simulink model "simuladorControlCuatrirrotor"  (Simulink 7.4)
settings: Solver=ode45  StartTime=0.0  StopTime=720  FixedStep=0.06  MaxStep=0.06  RelTol=1e-3
values from neighbouring files (symbols this model uses):
  radio = 0.1    [simulaControl.m]
  ruta = [0,0;ruta]    [pintascdata.m]    (also in pintascdata_tb2.m; simulaControl.m = [12 0;12 5;7 -5;-1 4;-6 -5;-2 0])
libraries: simulink x5
settings Model: Creator=xblasco  LastModifiedBy=xblasco

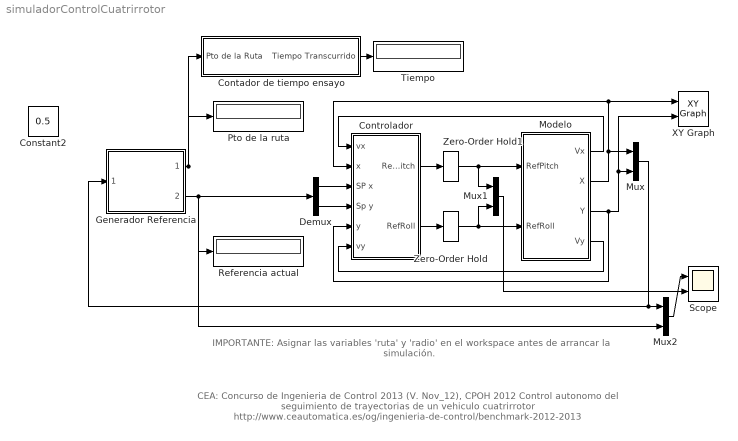
== system simuladorControlCuatrirrotor ==
  note: IMPORTANTE:
      | Asignar las variables 'ruta' y 'radio' en el workspace antes de arrancar la simulación.
  note: CEA: Concurso de Ingenieria de Control 2013 (V. Nov_12), CPOH 2012
      | Control autonomo del seguimiento de trayectorias de un vehiculo cuatrirrotor
      | http://www.ceautomatica.es/og/ingenieria-de-control/benchmark-2012-2013
  " Modelo" : Subsystem
  Contador de tiempo ensayo : Subsystem
  Controlador : Subsystem
  Demux : Demux  Outputs=2
  Generador Referencia : Subsystem
  Mux : Mux  Inputs=2
  Mux1 : Mux  Inputs=2
  Mux2 : Mux  Inputs=2
  Pto de la ruta : Display
  Referencia actual : Display
  Scope : Scope  NumInputPorts=2
      settings: YMin=-5~-1  YMax=15~1  SaveName=scdata  SampleInput=on  SampleTime=0.06
  Tiempo : Display
  XY Graph : simulink/Sinks/XY Graph  SystemSampleTime=-1  xmin=-10  xmax=15  ymin=-6  ymax=6  st=-1
  Zero-Order Hold : ZeroOrderHold  SampleTime=0.06
  Zero-Order Hold1 : ZeroOrderHold  SampleTime=0.06
  Constant2 : Constant  IOType=siggen  Value=0.5  OutDataType=sfix(16)  OutScaling=2^0
  wires:
  Generador Referencia/2(Siguiente pos) -> Referencia actual/1, Demux/1, Mux2/2
  Generador Referencia/1(Pto de la ruta) -> Pto de la ruta/1, Contador de tiempo ensayo/1(Pto de la Ruta)
  Controlador/1(RefPitch) -> Zero-Order Hold1/1
  Controlador/2(RefRoll) -> Zero-Order Hold/1
  Mux/1 -> Generador Referencia/1(Posicion  actual), Mux2/1
  Zero-Order Hold/1 -> " Modelo"/2(RefRoll), Mux1/2
  Zero-Order Hold1/1 -> " Modelo"/1(RefPitch), Mux1/1
  " Modelo"/2(X) -> Mux/1, XY Graph/1, Controlador/2(x)
  " Modelo"/3(Y) -> Controlador/5(y), XY Graph/2, Mux/2
  Mux1/1 -> Scope/2
  " Modelo"/1(Vx) -> Controlador/1(vx)
  Mux2/1 -> Scope/1
  Demux/1 -> Controlador/3(SP x)
  Demux/2 -> Controlador/4(Sp y)
  Contador de tiempo ensayo/1(Tiempo Transcurrido) -> Tiempo/1
  " Modelo"/4(Vy) -> Controlador/6(vy)

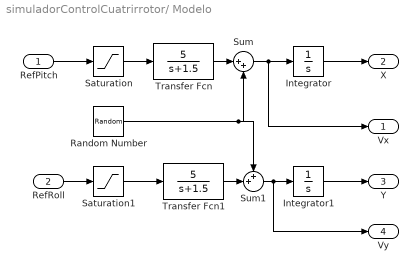
== system simuladorControlCuatrirrotor/ Modelo ==
  RefPitch : Inport  PortDimensions=1  SampleTime=0.06
  RefRoll : Inport  Port=2  PortDimensions=1  SampleTime=0.06
  Integrator : Integrator
  Integrator1 : Integrator
  Random Number : RandomNumber  Variance=0.3  SampleTime=0.06
  Saturation : Saturate  UpperLimit=1  LowerLimit=-1  OutDataType=fixdt(1, 16)  OutScaling=2^0
  Saturation1 : Saturate  UpperLimit=1  LowerLimit=-1  OutDataType=fixdt(1, 16)  OutScaling=2^0
  Sum : Sum  Inputs=|++  OutDataType=fixdt(1, 16)  OutScaling=2^0
  Sum1 : Sum  Inputs=++|  OutDataType=fixdt(1, 16)  OutScaling=2^0
  Transfer Fcn : TransferFcn  Numerator=[5]  Denominator=[1 1.5]
  Transfer Fcn1 : TransferFcn  Numerator=[5]  Denominator=[1 1.5]
  Vx : Outport
  X : Outport  Port=2
  Y : Outport  Port=3
  Vy : Outport  Port=4
  wires:
  RefPitch/1 -> Saturation/1
  RefRoll/1 -> Saturation1/1
  Integrator/1 -> X/1
  Integrator1/1 -> Y/1
  Saturation/1 -> Transfer Fcn/1
  Saturation1/1 -> Transfer Fcn1/1
  Transfer Fcn/1 -> Sum/1
  Sum/1 -> Integrator/1, Vx/1
  Random Number/1 -> Sum/2, Sum1/1
  Transfer Fcn1/1 -> Sum1/2
  Sum1/1 -> Integrator1/1, Vy/1

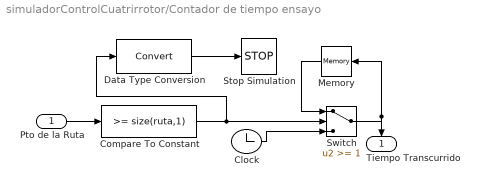
== system simuladorControlCuatrirrotor/Contador de tiempo ensayo ==
  Pto de la Ruta : Inport
  Clock : Clock
      settings: Decimation=10
  Compare To Constant : simulink/Logic and Bit Operations/Compare To Constant  SystemSampleTime=-1  relop=>=  const=size(ruta,1)  LogicOutDataTypeMode=uint8
  Data Type Conversion : DataTypeConversion  OutDataType=fixdt(1, 16)  OutScaling=2^0
  Memory : Memory
  Stop Simulation : Stop
  Switch : Switch  Threshold=1  OutDataType=fixdt(1, 16)  OutScaling=2^0
  Tiempo Transcurrido : Outport
  wires:
  Clock/1 -> Switch/3
  Compare To Constant/1 -> Switch/2, Data Type Conversion/1
  Switch/1 -> Memory/1, Tiempo Transcurrido/1
  Memory/1 -> Switch/1
  Data Type Conversion/1 -> Stop Simulation/1
  Pto de la Ruta/1 -> Compare To Constant/1

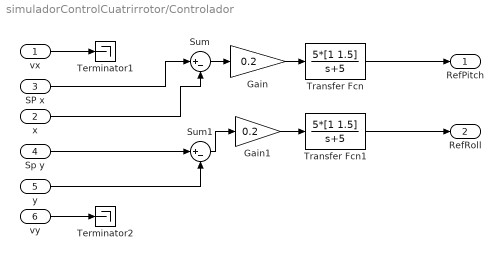
== system simuladorControlCuatrirrotor/Controlador ==
  vx : Inport
  x : Inport  Port=2
  SP x : Inport  Port=3
  Sp y : Inport  Port=4
  y : Inport  Port=5
  vy : Inport  Port=6
  Gain : Gain  Gain=0.2  ParameterDataType=fixdt(1, 16)  ParameterScaling=2^0  OutDataType=fixdt(1, 16)  OutScaling=2^0
  Gain1 : Gain  Gain=0.2  ParameterDataType=fixdt(1, 16)  ParameterScaling=2^0  OutDataType=fixdt(1, 16)  OutScaling=2^0
  Sum : Sum  Inputs=|+-  OutDataType=fixdt(1, 16)  OutScaling=2^0
  Sum1 : Sum  Inputs=|+-  OutDataType=fixdt(1, 16)  OutScaling=2^0
  Terminator1 : Terminator
  Terminator2 : Terminator
  Transfer Fcn : TransferFcn  Numerator=5*[1 1.5]  Denominator=[1 5]
  Transfer Fcn1 : TransferFcn  Numerator=5*[1 1.5]  Denominator=[1 5]
  RefPitch : Outport
  RefRoll : Outport  Port=2
  wires:
  Sum/1 -> Gain/1
  Sum1/1 -> Gain1/1
  Gain/1 -> Transfer Fcn/1
  Gain1/1 -> Transfer Fcn1/1
  Transfer Fcn/1 -> RefPitch/1
  Transfer Fcn1/1 -> RefRoll/1
  x/1 -> Sum/2
  SP x/1 -> Sum/1
  vx/1 -> Terminator1/1
  vy/1 -> Terminator2/1
  y/1 -> Sum1/2
  Sp y/1 -> Sum1/1

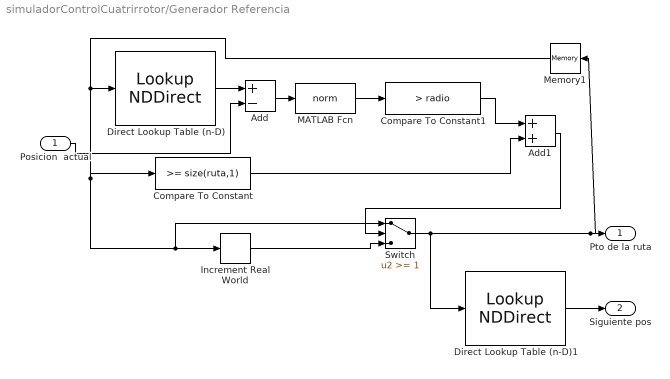
== system simuladorControlCuatrirrotor/Generador Referencia ==
  Posicion  actual : Inport
  Add : Sum  Inputs=+-  OutDataType=fixdt(1, 16)  OutScaling=2^-10
  Add1 : Sum  OutDataType=fixdt(1, 16)  OutScaling=2^-10
  Compare To Constant : simulink/Logic and Bit Operations/Compare To Constant  SystemSampleTime=-1  relop=>=  const=size(ruta,1)  LogicOutDataTypeMode=uint8
  Compare To Constant1 : simulink/Logic and Bit Operations/Compare To Constant  SystemSampleTime=-1  relop=>  const=radio  LogicOutDataTypeMode=uint8
  Direct Lookup Table (n-D) : LookupNDDirect  InputsSelectThisObjectFromTable=Column  Table=ruta'
  Direct Lookup Table (n-D)1 : LookupNDDirect  InputsSelectThisObjectFromTable=Column  Table=ruta'
  Increment Real World : simulink/Additional Math & Discrete/Additional Math: Increment - Decrement/Increment Real World  SystemSampleTime=-1
  MATLAB Fcn : MATLABFcn  MATLABFcn=norm  Output1D=off
  Memory1 : Memory
  Switch : Switch  Threshold=1  OutDataType=fixdt(1, 16)  OutScaling=2^0
  Pto de la ruta : Outport
  Siguiente pos : Outport  Port=2
  wires:
  Direct Lookup Table (n-D)/1 -> Add/1
  Add/1 -> MATLAB Fcn/1
  Increment Real World/1 -> Switch/3
  Switch/1 -> Direct Lookup Table (n-D)1/1, Pto de la ruta/1, Memory1/1
  Posicion  actual/1 -> Add/2
  Direct Lookup Table (n-D)1/1 -> Siguiente pos/1
  MATLAB Fcn/1 -> Compare To Constant1/1
  Compare To Constant1/1 -> Add1/1
  Compare To Constant/1 -> Add1/2
  Add1/1 -> Switch/2
  Memory1/1 -> Direct Lookup Table (n-D)/1, Compare To Constant/1, Switch/1, Increment Real World/1
